simulink library "qrd_matrix_library"  (Simulink 8.7)
settings: Solver=ode45  StartTime=0.0  StopTime=10.0  RelTol=1e-3
values from neighbouring files (symbols this model uses):
  vectorization = 2    [qrd_test.m]
undefined symbols (not defined in the file or in its folder): AdvDSPBChannelOutDisplay, AdvDSPBDMemDisplay, Back_Substitution_instances, column_count, column_count_1, column_count_2, dpoly, dspba_ChannelInVis, dspba_ChannelOutVis, dspba_internal_get_channel_ports, evalAionMaskParam, latency, primtype, QRD_vectorization, recipsqrt, row, row_count, row_count_1, row_count_2, UseDontCare, value, x
libraries: DSPBAPrim x683, DSPBAControl x37, qrd_matrix_library x33, DSPBAVectorUtil x6, DSPBAVectorPrim x3
(part 2 of 8)

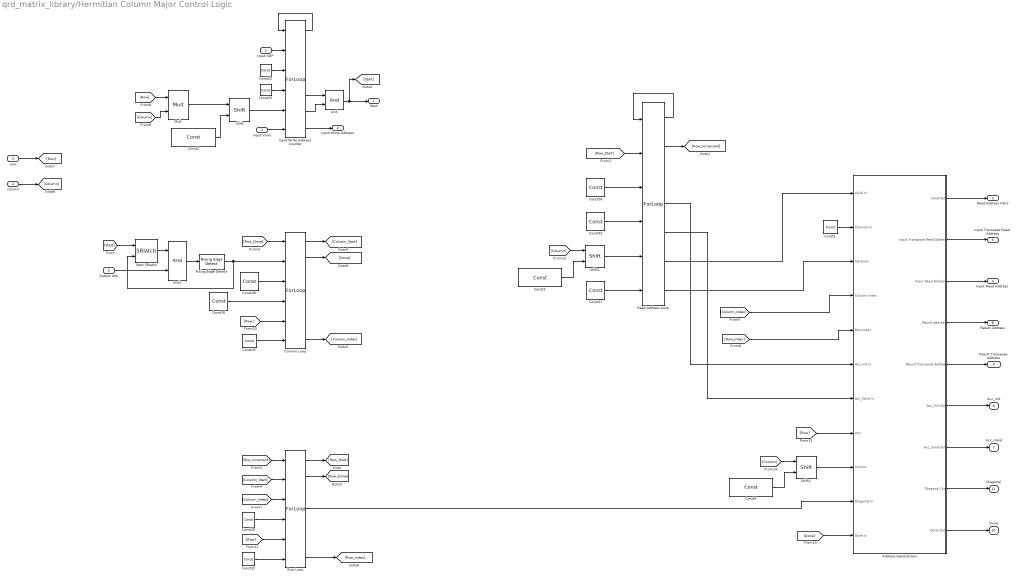
== system qrd_matrix_library/Hermitian Column Major Control Logic ==
  Input Valid : Inport
  Input SOP : Inport  Port=2
  row : Inport  Port=3
  column : Inport  Port=4
  Output Idle : Inport  Port=5
  Address Generatioon : Subsystem
  And : DSPBAPrim/And  primtype=and  nInputs=2  nOutputs=1  omode=Inherit via internal rule  otype=sfix(16)  scale=2^-15  rndmethod=Unbiased  factor=1  satmethod=Symmetric  shift_vec=[0 1 2 -1]  value=0  inPortNames=[' '; ' '; ' '; ' '; ' '; ' '; ' '; ' '; ' '; ' '; ' '; ' '; ' '; ' '; ' '; ' '; ]  outPortNames=[' ']  dspbaimage=dspba_prim.jpg  text=fprintf('&');  style=Optimised  visibilities=8+2  version=20090407
  And1 : DSPBAPrim/And  primtype=and  nInputs=2  nOutputs=1  omode=Inherit via internal rule  otype=sfix(16)  scale=2^-15  rndmethod=Unbiased  factor=1  satmethod=Symmetric  shift_vec=[0 1 2 -1]  value=0  inPortNames=[' '; ' '; ' '; ' '; ' '; ' '; ' '; ' '; ' '; ' '; ' '; ' '; ' '; ' '; ' '; ' '; ]  outPortNames=[' ']  dspbaimage=dspba_prim.jpg  text=fprintf('&');  style=Optimised  visibilities=8+2  version=20090407
  Column Loop : DSPBAPrim/ForLoop  looptest=<
  Const1 : DSPBAPrim/Const  primtype=const  nInputs=0  nOutputs=1  omode=Specify via dialog  otype=uint(8)  scale=1  rndmethod=Unbiased  factor=1  satmethod=Symmetric  shift_vec=[0 1 2 -1]  value=0  inPortNames=['+'; '+';]  outPortNames=[' ']  dspbaimage=dspba_prim.jpg  text=fprintf('%s', num2str(value));  style=Optimised  visibilities=8 + 1024  floatPrecision=float32_m23  version=20120820
  Const2 : DSPBAPrim/Const  primtype=const  nInputs=0  nOutputs=1  omode=Inherit via internal rule  otype=uint(8)  scale=1  rndmethod=Unbiased  factor=1  satmethod=Symmetric  shift_vec=[0 1 2 -1]  value=nextpow2(vectorization)  inPortNames=['+'; '+';]  outPortNames=[' ']  dspbaimage=dspba_prim.jpg  text=fprintf('%s', num2str(value));  style=Optimised  visibilities=8 + 1024  floatPrecision=float32_m23  version=20120820
  Const{23,26,29,33,35,37} (6 alike) : DSPBAPrim/Const  primtype=const  nInputs=0  nOutputs=1  omode=Inherit via internal rule  otype=uint(8)  scale=1  rndmethod=Unbiased  factor=1  satmethod=Symmetric  shift_vec=[0 1 2 -1]  value=1  inPortNames=['+'; '+';]  outPortNames=[' ']  dspbaimage=dspba_prim.jpg  text=fprintf('%s', num2str(value));  style=Optimised  visibilities=8 + 1024  floatPrecision=float32_m23  version=20120820
  Const25 : DSPBAPrim/Const  primtype=const  nInputs=0  nOutputs=1  omode=Inherit via internal rule  otype=uint(8)  scale=1  rndmethod=Unbiased  factor=1  satmethod=Symmetric  shift_vec=[0 1 2 -1]  value=0  inPortNames=['+'; '+';]  outPortNames=[' ']  dspbaimage=dspba_prim.jpg  text=fprintf('%s', num2str(value));  style=Optimised  visibilities=8 + 1024  floatPrecision=float32_m23  version=20120820
  Const28 : DSPBAPrim/Const  primtype=const  nInputs=0  nOutputs=1  omode=Inherit via internal rule  otype=uint(8)  scale=1  rndmethod=Unbiased  factor=1  satmethod=Symmetric  shift_vec=[0 1 2 -1]  value=0  inPortNames=['+'; '+';]  outPortNames=[' ']  dspbaimage=dspba_prim.jpg  text=fprintf('%s', num2str(value));  style=Optimised  visibilities=8 + 1024  floatPrecision=float32_m23  version=20120820
  Const3 : DSPBAPrim/Const  primtype=const  nInputs=0  nOutputs=1  omode=Inherit via internal rule  otype=uint(8)  scale=1  rndmethod=Unbiased  factor=1  satmethod=Symmetric  shift_vec=[0 1 2 -1]  value=nextpow2(vectorization)  inPortNames=['+'; '+';]  outPortNames=[' ']  dspbaimage=dspba_prim.jpg  text=fprintf('%s', num2str(value));  style=Optimised  visibilities=8 + 1024  floatPrecision=float32_m23  version=20120820
  Const32 : DSPBAPrim/Const  primtype=const  nInputs=0  nOutputs=1  omode=boolean  otype=uint(8)  scale=1  rndmethod=Unbiased  factor=1  satmethod=Symmetric  shift_vec=[0 1 2 -1]  value=1  inPortNames=['+'; '+';]  outPortNames=[' ']  dspbaimage=dspba_prim.jpg  text=fprintf('%s', num2str(value));  style=Optimised  visibilities=8 + 1024  floatPrecision=float32_m23  version=20120820
  Const36 : DSPBAPrim/Const  primtype=const  nInputs=0  nOutputs=1  omode=Inherit via internal rule  otype=uint(8)  scale=1  rndmethod=Unbiased  factor=1  satmethod=Symmetric  shift_vec=[0 1 2 -1]  value=0  inPortNames=['+'; '+';]  outPortNames=[' ']  dspbaimage=dspba_prim.jpg  text=fprintf('%s', num2str(value));  style=Optimised  visibilities=8 + 1024  floatPrecision=float32_m23  version=20120820
  Const4 : DSPBAPrim/Const  primtype=const  nInputs=0  nOutputs=1  omode=Inherit via internal rule  otype=uint(8)  scale=1  rndmethod=Unbiased  factor=1  satmethod=Symmetric  shift_vec=[0 1 2 -1]  value=nextpow2(vectorization)  inPortNames=['+'; '+';]  outPortNames=[' ']  dspbaimage=dspba_prim.jpg  text=fprintf('%s', num2str(value));  style=Optimised  visibilities=8 + 1024  floatPrecision=float32_m23  version=20120820
  Input Write Address Counter : DSPBAPrim/ForLoop  looptest=<
  Mult : DSPBAPrim/Mult  primtype=mult  nInputs=2  nOutputs=1  omode=Inherit via internal rule  otype=sfix(16)  scale=2^-15  rndmethod=Unbiased  factor=1  satmethod=Symmetric  shift_vec=[0 1 2 -1]  value=0  inPortNames=[' '; ' ';]  outPortNames=[' ']  dspbaimage=dspba_prim.jpg  text=fprintf('X');  style=Optimised  visibilities=8+2^18+2^19  floatPrecision=float32_m23  floatRounding=correct  advOptions=[]  version=20130115
  Read Address Loop : DSPBAPrim/ForLoop  looptest=<
  Rising Edge Detect : qrd_matrix_library/hermitian_matrix_multiplication/Rising Edge Detect
  Row Loop : DSPBAPrim/ForLoop  looptest=<
  Shift : DSPBAPrim/Shift  primtype=shift  nInputs=2  nOutputs=1  omode=Inherit via internal rule  otype=sfix(16)  scale=2^-15  rndmethod=Unbiased  factor=1  satmethod=Symmetric  shift_vec=[0 1 2 -1]  value=0  inPortNames=['a'; 'b';]  outPortNames=[' ']  dspbaimage=dspba_prim.jpg  text=fprintf('a >> b');  style=Optimised  visibilities=8  version=20090407
  Shift1 : DSPBAPrim/Shift  primtype=shift  nInputs=2  nOutputs=1  omode=Inherit via internal rule  otype=sfix(16)  scale=2^-15  rndmethod=Unbiased  factor=1  satmethod=Symmetric  shift_vec=[0 1 2 -1]  value=0  inPortNames=['a'; 'b';]  outPortNames=[' ']  dspbaimage=dspba_prim.jpg  text=fprintf('a >> b');  style=Optimised  visibilities=8  version=20090407
  Shift2 : DSPBAPrim/Shift  primtype=shift  nInputs=2  nOutputs=1  omode=Inherit via internal rule  otype=sfix(16)  scale=2^-15  rndmethod=Unbiased  factor=1  satmethod=Symmetric  shift_vec=[0 1 2 -1]  value=0  inPortNames=['a'; 'b';]  outPortNames=[' ']  dspbaimage=dspba_prim.jpg  text=fprintf('a >> b');  style=Optimised  visibilities=8  version=20090407
  Start SRlatch : DSPBAControl/SRlatch
  Start : Outport
  Input Write Address : Outport  Port=2
  Read Address Valid : Outport  Port=3
  Input Read Address : Outport  Port=4
  Input Transpose Read Address : Outport  Port=5
  Acc_Init : Outport  Port=6
  Acc_Valid : Outport  Port=7
  Result Address : Outport  Port=8
  Result Transpose Address : Outport  Port=9
  Done : Outport  Port=10
  Diagonal : Outport  Port=11
  wires:
  Address Generatioon/9(Done Out) -> Done/1
  [Done] -> Address Generatioon/11(Done In)
  [Row_Start] -> Read Address Loop/2
  Input SOP/1 -> Input Write Address Counter/2
  Read Address Loop/2 -> [Row_Increment]
  Input Write Address Counter/6 -> And/2
  Input Write Address Counter/5 -> And/1
  And/1 -> Start/1, [Start]
  Input Write Address Counter/1 -> Input Write Address Counter/1
  Input Valid/1 -> Input Write Address Counter/6
  Shift2/1 -> Address Generatioon/9(column)
  Const4/1 -> Shift2/2
  [Column] -> Shift2/1
  [Row] -> Address Generatioon/8(row)
  Const3/1 -> Shift1/2
  [Column] -> Shift1/1
  Const2/1 -> Shift/2
  Mult/1 -> Shift/1
  [Column] -> Mult/2
  [Row] -> Mult/1
  column/1 -> [Column]
  row/1 -> [Row]
  Address Generatioon/8(Diagonal Out) -> Diagonal/1
  Row Loop/4 -> Address Generatioon/10(Diagonal In)
  Const1/1 -> Address Generatioon/2(Channel In)
  Address Generatioon/6(Acc_Init Out) -> Acc_Init/1
  Address Generatioon/7(Acc_Valid Out) -> Acc_Valid/1
  Read Address Loop/6 -> Address Generatioon/1(Valid In)
  Address Generatioon/5(Result Transpose Address) -> Result Transpose Address/1
  Address Generatioon/4(Result Address) -> Result Address/1
  Address Generatioon/3(Input Read Address) -> Input Read Address/1
  Address Generatioon/2(Input Transpose Read Address) -> Input Transpose Read Address/1
  [Row_Index] -> Address Generatioon/5(Row Index)
  [Column_Index] -> Address Generatioon/4(Column Index)
  Read Address Loop/7 -> Address Generatioon/3(Iteration)
  Column Loop/2 -> [Done]
  Read Address Loop/5 -> Address Generatioon/7(Acc_Valid In)
  Read Address Loop/4 -> Address Generatioon/6(Acc_Init In)
  Address Generatioon/1(Valid Out) -> Read Address Valid/1
  Row Loop/7 -> [Row_Index]
  Const37/1 -> Read Address Loop/6
  Column Loop/1 -> [Column_Start]
  [Column_Start] -> Row Loop/2
  [Row_Done] -> Column Loop/1
  Row Loop/2 -> [Row_Done]
  [Row_Increment] -> Row Loop/1
  Row Loop/1 -> [Row_Start]
  Const35/1 -> Column Loop/6
  Const32/1 -> Row Loop/6
  Shift1/1 -> Read Address Loop/5
  Const33/1 -> Read Address Loop/4
  Const36/1 -> Read Address Loop/3
  Read Address Loop/1 -> Read Address Loop/1
  Column Loop/7 -> [Column_Index]
  [Column_Index] -> Row Loop/3
  Const29/1 -> Row Loop/4
  [Row] -> Row Loop/5
  Const28/1 -> Column Loop/3
  Const26/1 -> Column Loop/4
  [Row] -> Column Loop/5
  Input Write Address Counter/7 -> Input Write Address/1
  Const25/1 -> Input Write Address Counter/3
  Const23/1 -> Input Write Address Counter/4
  Shift/1 -> Input Write Address Counter/5
  [Start] -> Start SRlatch/1
  Start SRlatch/1 -> And1/1
  Output Idle/1 -> And1/2
  And1/1 -> Rising Edge Detect/1
  Rising Edge Detect/1 -> Column Loop/2, Start SRlatch/2

== system qrd_matrix_library/Hermitian Control Logic ==
  Input Valid : Inport
  Input SOP : Inport  Port=2
  row : Inport  Port=3
  column : Inport  Port=4
  Hermitian Column Major Control Logic : qrd_matrix_library/Hermitian Column Major Control Logic
  Start : Outport
  Input Write Address : Outport  Port=2
  Read Address Valid : Outport  Port=3
  Input Read Address : Outport  Port=4
  Input Transpose Read Address : Outport  Port=5
  Acc_Init : Outport  Port=6
  Acc_Valid : Outport  Port=7
  Result Address : Outport  Port=8
  Result Transpose Address : Outport  Port=9
  Done : Outport  Port=10
  Diagonal : Outport  Port=11
  wires:
  Input Valid/1 -> Hermitian Column Major Control Logic/1
  Input SOP/1 -> Hermitian Column Major Control Logic/2
  row/1 -> Hermitian Column Major Control Logic/3
  column/1 -> Hermitian Column Major Control Logic/4
  Hermitian Column Major Control Logic/1 -> Start/1
  Hermitian Column Major Control Logic/2 -> Input Write Address/1
  Hermitian Column Major Control Logic/3 -> Read Address Valid/1
  Hermitian Column Major Control Logic/4 -> Input Read Address/1
  Hermitian Column Major Control Logic/5 -> Input Transpose Read Address/1
  Hermitian Column Major Control Logic/6 -> Acc_Init/1
  Hermitian Column Major Control Logic/7 -> Acc_Valid/1
  Hermitian Column Major Control Logic/8 -> Result Address/1
  Hermitian Column Major Control Logic/9 -> Result Transpose Address/1
  Hermitian Column Major Control Logic/10 -> Done/1
  Hermitian Column Major Control Logic/11 -> Diagonal/1

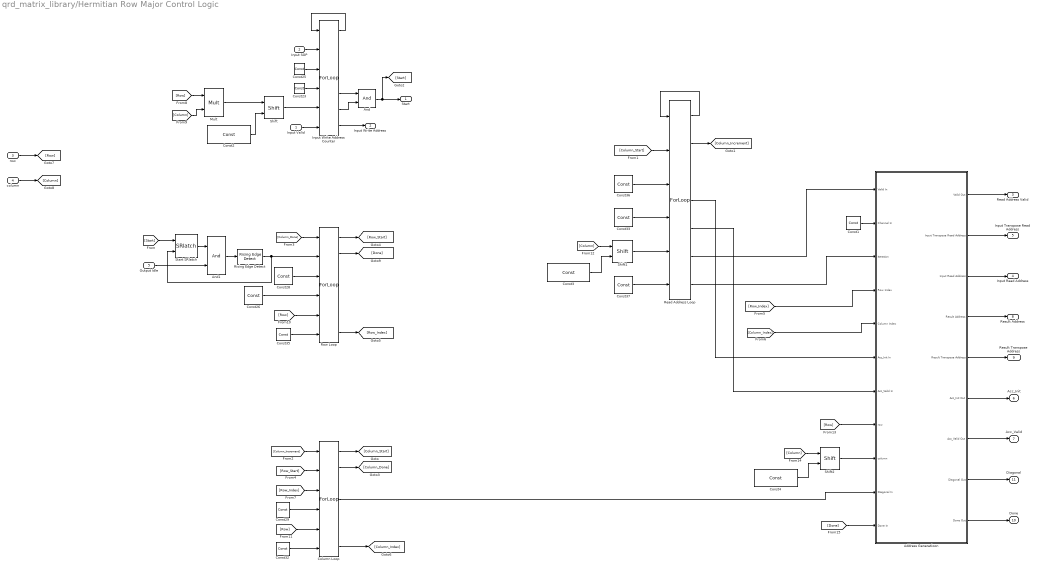
== system qrd_matrix_library/Hermitian Row Major Control Logic ==
  Input Valid : Inport
  Input SOP : Inport  Port=2
  row : Inport  Port=3
  column : Inport  Port=4
  Output Idle : Inport  Port=5
  Address Generatioon : Subsystem
  And : DSPBAPrim/And  primtype=and  nInputs=2  nOutputs=1  omode=Inherit via internal rule  otype=sfix(16)  scale=2^-15  rndmethod=Unbiased  factor=1  satmethod=Symmetric  shift_vec=[0 1 2 -1]  value=0  inPortNames=[' '; ' '; ' '; ' '; ' '; ' '; ' '; ' '; ' '; ' '; ' '; ' '; ' '; ' '; ' '; ' '; ]  outPortNames=[' ']  dspbaimage=dspba_prim.jpg  text=fprintf('&');  style=Optimised  visibilities=8+2  version=20090407
  And1 : DSPBAPrim/And  primtype=and  nInputs=2  nOutputs=1  omode=Inherit via internal rule  otype=sfix(16)  scale=2^-15  rndmethod=Unbiased  factor=1  satmethod=Symmetric  shift_vec=[0 1 2 -1]  value=0  inPortNames=[' '; ' '; ' '; ' '; ' '; ' '; ' '; ' '; ' '; ' '; ' '; ' '; ' '; ' '; ' '; ' '; ]  outPortNames=[' ']  dspbaimage=dspba_prim.jpg  text=fprintf('&');  style=Optimised  visibilities=8+2  version=20090407
  Column Loop : DSPBAPrim/ForLoop  looptest=<
  Const1 : DSPBAPrim/Const  primtype=const  nInputs=0  nOutputs=1  omode=Specify via dialog  otype=uint(8)  scale=1  rndmethod=Unbiased  factor=1  satmethod=Symmetric  shift_vec=[0 1 2 -1]  value=0  inPortNames=['+'; '+';]  outPortNames=[' ']  dspbaimage=dspba_prim.jpg  text=fprintf('%s', num2str(value));  style=Optimised  visibilities=8 + 1024  floatPrecision=float32_m23  version=20120820
  Const2 : DSPBAPrim/Const  primtype=const  nInputs=0  nOutputs=1  omode=Inherit via internal rule  otype=uint(8)  scale=1  rndmethod=Unbiased  factor=1  satmethod=Symmetric  shift_vec=[0 1 2 -1]  value=nextpow2(vectorization)  inPortNames=['+'; '+';]  outPortNames=[' ']  dspbaimage=dspba_prim.jpg  text=fprintf('%s', num2str(value));  style=Optimised  visibilities=8 + 1024  floatPrecision=float32_m23  version=20120820
  Const{23,26,29,33,35,37} (6 alike) : DSPBAPrim/Const  primtype=const  nInputs=0  nOutputs=1  omode=Inherit via internal rule  otype=uint(8)  scale=1  rndmethod=Unbiased  factor=1  satmethod=Symmetric  shift_vec=[0 1 2 -1]  value=1  inPortNames=['+'; '+';]  outPortNames=[' ']  dspbaimage=dspba_prim.jpg  text=fprintf('%s', num2str(value));  style=Optimised  visibilities=8 + 1024  floatPrecision=float32_m23  version=20120820
  Const25 : DSPBAPrim/Const  primtype=const  nInputs=0  nOutputs=1  omode=Inherit via internal rule  otype=uint(8)  scale=1  rndmethod=Unbiased  factor=1  satmethod=Symmetric  shift_vec=[0 1 2 -1]  value=0  inPortNames=['+'; '+';]  outPortNames=[' ']  dspbaimage=dspba_prim.jpg  text=fprintf('%s', num2str(value));  style=Optimised  visibilities=8 + 1024  floatPrecision=float32_m23  version=20120820
  Const28 : DSPBAPrim/Const  primtype=const  nInputs=0  nOutputs=1  omode=Inherit via internal rule  otype=uint(8)  scale=1  rndmethod=Unbiased  factor=1  satmethod=Symmetric  shift_vec=[0 1 2 -1]  value=0  inPortNames=['+'; '+';]  outPortNames=[' ']  dspbaimage=dspba_prim.jpg  text=fprintf('%s', num2str(value));  style=Optimised  visibilities=8 + 1024  floatPrecision=float32_m23  version=20120820
  Const3 : DSPBAPrim/Const  primtype=const  nInputs=0  nOutputs=1  omode=Inherit via internal rule  otype=uint(8)  scale=1  rndmethod=Unbiased  factor=1  satmethod=Symmetric  shift_vec=[0 1 2 -1]  value=nextpow2(vectorization)  inPortNames=['+'; '+';]  outPortNames=[' ']  dspbaimage=dspba_prim.jpg  text=fprintf('%s', num2str(value));  style=Optimised  visibilities=8 + 1024  floatPrecision=float32_m23  version=20120820
  Const32 : DSPBAPrim/Const  primtype=const  nInputs=0  nOutputs=1  omode=boolean  otype=uint(8)  scale=1  rndmethod=Unbiased  factor=1  satmethod=Symmetric  shift_vec=[0 1 2 -1]  value=1  inPortNames=['+'; '+';]  outPortNames=[' ']  dspbaimage=dspba_prim.jpg  text=fprintf('%s', num2str(value));  style=Optimised  visibilities=8 + 1024  floatPrecision=float32_m23  version=20120820
  Const36 : DSPBAPrim/Const  primtype=const  nInputs=0  nOutputs=1  omode=Inherit via internal rule  otype=uint(8)  scale=1  rndmethod=Unbiased  factor=1  satmethod=Symmetric  shift_vec=[0 1 2 -1]  value=0  inPortNames=['+'; '+';]  outPortNames=[' ']  dspbaimage=dspba_prim.jpg  text=fprintf('%s', num2str(value));  style=Optimised  visibilities=8 + 1024  floatPrecision=float32_m23  version=20120820
  Const4 : DSPBAPrim/Const  primtype=const  nInputs=0  nOutputs=1  omode=Inherit via internal rule  otype=uint(8)  scale=1  rndmethod=Unbiased  factor=1  satmethod=Symmetric  shift_vec=[0 1 2 -1]  value=nextpow2(vectorization)  inPortNames=['+'; '+';]  outPortNames=[' ']  dspbaimage=dspba_prim.jpg  text=fprintf('%s', num2str(value));  style=Optimised  visibilities=8 + 1024  floatPrecision=float32_m23  version=20120820
  Input Write Address Counter : DSPBAPrim/ForLoop  looptest=<
  Mult : DSPBAPrim/Mult  primtype=mult  nInputs=2  nOutputs=1  omode=Inherit via internal rule  otype=sfix(16)  scale=2^-15  rndmethod=Unbiased  factor=1  satmethod=Symmetric  shift_vec=[0 1 2 -1]  value=0  inPortNames=[' '; ' ';]  outPortNames=[' ']  dspbaimage=dspba_prim.jpg  text=fprintf('X');  style=Optimised  visibilities=8+2^18+2^19  floatPrecision=float32_m23  floatRounding=correct  advOptions=[]  version=20130115
  Read Address Loop : DSPBAPrim/ForLoop  looptest=<
  Rising Edge Detect : qrd_matrix_library/hermitian_matrix_multiplication/Rising Edge Detect
  Row Loop : DSPBAPrim/ForLoop  looptest=<
  Shift : DSPBAPrim/Shift  primtype=shift  nInputs=2  nOutputs=1  omode=Inherit via internal rule  otype=sfix(16)  scale=2^-15  rndmethod=Unbiased  factor=1  satmethod=Symmetric  shift_vec=[0 1 2 -1]  value=0  inPortNames=['a'; 'b';]  outPortNames=[' ']  dspbaimage=dspba_prim.jpg  text=fprintf('a >> b');  style=Optimised  visibilities=8  version=20090407
  Shift1 : DSPBAPrim/Shift  primtype=shift  nInputs=2  nOutputs=1  omode=Inherit via internal rule  otype=sfix(16)  scale=2^-15  rndmethod=Unbiased  factor=1  satmethod=Symmetric  shift_vec=[0 1 2 -1]  value=0  inPortNames=['a'; 'b';]  outPortNames=[' ']  dspbaimage=dspba_prim.jpg  text=fprintf('a >> b');  style=Optimised  visibilities=8  version=20090407
  Shift2 : DSPBAPrim/Shift  primtype=shift  nInputs=2  nOutputs=1  omode=Inherit via internal rule  otype=sfix(16)  scale=2^-15  rndmethod=Unbiased  factor=1  satmethod=Symmetric  shift_vec=[0 1 2 -1]  value=0  inPortNames=['a'; 'b';]  outPortNames=[' ']  dspbaimage=dspba_prim.jpg  text=fprintf('a >> b');  style=Optimised  visibilities=8  version=20090407
  Start SRlatch : DSPBAControl/SRlatch
  Start : Outport
  Input Write Address : Outport  Port=2
  Read Address Valid : Outport  Port=3
  Input Read Address : Outport  Port=4
  Input Transpose Read Address : Outport  Port=5
  Acc_Init : Outport  Port=6
  Acc_Valid : Outport  Port=7
  Result Address : Outport  Port=8
  Result Transpose Address : Outport  Port=9
  Done : Outport  Port=10
  Diagonal : Outport  Port=11
  wires:
  Address Generatioon/9(Done Out) -> Done/1
  [Done] -> Address Generatioon/11(Done In)
  [Column_Start] -> Read Address Loop/2
  Input SOP/1 -> Input Write Address Counter/2
  Read Address Loop/2 -> [Column_Increment]
  Input Write Address Counter/6 -> And/2
  Input Write Address Counter/5 -> And/1
  And/1 -> Start/1, [Start]
  Input Write Address Counter/1 -> Input Write Address Counter/1
  Input Valid/1 -> Input Write Address Counter/6
  Shift2/1 -> Address Generatioon/9(column)
  Const4/1 -> Shift2/2
  [Column] -> Shift2/1
  [Row] -> Address Generatioon/8(row)
  Const3/1 -> Shift1/2
  [Column] -> Shift1/1
  Const2/1 -> Shift/2
  Mult/1 -> Shift/1
  [Column] -> Mult/2
  [Row] -> Mult/1
  column/1 -> [Column]
  row/1 -> [Row]
  Address Generatioon/8(Diagonal Out) -> Diagonal/1
  Column Loop/4 -> Address Generatioon/10(Diagonal In)
  Const1/1 -> Address Generatioon/2(Channel In)
  Address Generatioon/6(Acc_Init Out) -> Acc_Init/1
  Address Generatioon/7(Acc_Valid Out) -> Acc_Valid/1
  Read Address Loop/6 -> Address Generatioon/1(Valid In)
  Address Generatioon/5(Result Transpose Address) -> Result Transpose Address/1
  Address Generatioon/4(Result Address) -> Result Address/1
  Address Generatioon/3(Input Read Address) -> Input Read Address/1
  Address Generatioon/2(Input Transpose Read Address) -> Input Transpose Read Address/1
  [Column_Index] -> Address Generatioon/5(Column Index)
  [Row_Index] -> Address Generatioon/4(Row Index)
  Read Address Loop/7 -> Address Generatioon/3(Iteration)
  Row Loop/2 -> [Done]
  Read Address Loop/5 -> Address Generatioon/7(Acc_Valid In)
  Read Address Loop/4 -> Address Generatioon/6(Acc_Init In)
  Address Generatioon/1(Valid Out) -> Read Address Valid/1
  Column Loop/7 -> [Column_Index]
  Const37/1 -> Read Address Loop/6
  Row Loop/1 -> [Row_Start]
  [Row_Start] -> Column Loop/2
  [Column_Done] -> Row Loop/1
  Column Loop/2 -> [Column_Done]
  [Column_Increment] -> Column Loop/1
  Column Loop/1 -> [Column_Start]
  Const35/1 -> Row Loop/6
  Const32/1 -> Column Loop/6
  Shift1/1 -> Read Address Loop/5
  Const33/1 -> Read Address Loop/4
  Const36/1 -> Read Address Loop/3
  Read Address Loop/1 -> Read Address Loop/1
  Row Loop/7 -> [Row_Index]
  [Start] -> Start SRlatch/1
  [Row_Index] -> Column Loop/3
  Const29/1 -> Column Loop/4
  [Row] -> Column Loop/5
  Const28/1 -> Row Loop/3
  Const26/1 -> Row Loop/4
  [Row] -> Row Loop/5
  Input Write Address Counter/7 -> Input Write Address/1
  Const25/1 -> Input Write Address Counter/3
  Const23/1 -> Input Write Address Counter/4
  Shift/1 -> Input Write Address Counter/5
  Start SRlatch/1 -> And1/1
  Output Idle/1 -> And1/2
  And1/1 -> Rising Edge Detect/1
  Rising Edge Detect/1 -> Start SRlatch/2, Row Loop/2

== system qrd_matrix_library/Latch ==
  Valid_In : Inport
  Channel_In : Inport  Port=2
  Data_In : Inport  Port=3
  ChannelIn : DSPBAPrim/ChannelIn  primtype=channelin  nInputs=dspba_internal_get_channel_ports(gcb)  nOutputs=dspba_internal_get_channel_ports(gcb)  omode=Inherit via internal rule  otype=sfix(16)  scale=2^-15  rndmethod=Unbiased  factor=1  satmethod=Symmetric  shift_vec=[0 1 2 -1]  value=1  inPortNames=['v'; 'c'; '0'; '1'; '2'; '3'; '4'; '5'; '6'; '7'; '8'; '9'; 'A'; 'B'; 'D'; 'E'; 'F'; 'G'; 'H'; 'I'; 'J'; 'K'; 'L'; 'M'; 'N'; 'O'; 'P'; 'Q'; 'R'; 'S'; 'T'; 'U'; 'W'; 'X'; 'Y'; 'Z']  outPortNames=['v'; 'c'; '0'; '1'; '2'; '3'; '4'; '5'; '6'; '7'; '8'; '9'; 'A'; 'B'; 'D'; 'E'; 'F'; 'G'; 'H'; 'I'; 'J'; 'K'; 'L'; 'M'; 'N'; 'O'; 'P'; 'Q'; 'R'; 'S'; 'T'; 'U'; 'W'; 'X'; 'Y'; 'Z']  dspbaimage=dspba_prim.jpg  text=fprintf('In');  style=Optimised  dataSignals=1  foldingEnabled=off  channels=1  sampleRate=200  packetBeginPresent=off  packetBeginEnabled=off  visibilities=dspba_ChannelInVis(gcb)  latencyCorrection=0  version=20141013
  ChannelOut : DSPBAPrim/ChannelOut  primtype=channelout  nInputs=dspba_internal_get_channel_ports(gcb)  nOutputs=dspba_internal_get_channel_ports(gcb)  omode=Inherit via internal rule  otype=sfix(16)  scale=2^-15  rndmethod=Unbiased  factor=1  satmethod=Symmetric  shift_vec=[0 1 2 -1]  value=1  inPortNames=['v'; 'c'; '0'; '1'; '2'; '3'; '4'; '5'; '6'; '7'; '8'; '9'; 'A'; 'B'; 'D'; 'E'; 'F'; 'G'; 'H'; 'I'; 'J'; 'K'; 'L'; 'M'; 'N'; 'O'; 'P'; 'Q'; 'R'; 'S'; 'T'; 'U'; 'W'; 'X'; 'Y'; 'Z']  outPortNames=['v'; 'c'; '0'; '1'; '2'; '3'; '4'; '5'; '6'; '7'; '8'; '9'; 'A'; 'B'; 'D'; 'E'; 'F'; 'G'; 'H'; 'I'; 'J'; 'K'; 'L'; 'M'; 'N'; 'O'; 'P'; 'Q'; 'R'; 'S'; 'T'; 'U'; 'W'; 'X'; 'Y'; 'Z']  dspbaimage=dspba_prim.jpg  text=fprintf('Out%s', AdvDSPBChannelOutDisplay(latency));  style=Optimised  dataSignals=1  foldingEnabled=off  channels=1  sampleRate=200  packetBeginPresent=off  packetBeginEnabled=off  visibilities=dspba_ChannelOutVis(gcb)  latency=0  latencyCorrection=0  version=20141013
  SynthesisInfo : DSPBAPrim/SynthesisInfo  primtype=synthinfo  nInputs=0  nOutputs=0  omode=Inherit via internal rule  otype=sfix(16)  scale=2^-15  rndmethod=Truncate  factor=1  satmethod=Symmetric  shift_vec=[0 1 2 -1]  value=99  inPortNames=[' '; ' ';]  outPortNames=[' ']  dspbaimage=dspba_prim_ctrl.jpg  text=fprintf('Style=%s', style);  style=Scheduled  visibilities=32768  constraintInUse=off  constraintRelation=>  constraintLimit=2  bitAccurate=off  version=20150220
  latch_0L : DSPBAControl/latch_0L
  Valid_Out : Outport
  Channel_Out : Outport  Port=2
  Data_Out : Outport  Port=3
  wires:
  Valid_In/1 -> ChannelIn/1
  Data_In/1 -> ChannelIn/3
  Channel_In/1 -> ChannelIn/2
  ChannelIn/1 -> ChannelOut/1, latch_0L/1
  latch_0L/1 -> ChannelOut/3
  ChannelIn/2 -> ChannelOut/2
  ChannelIn/3 -> latch_0L/2
  ChannelOut/1 -> Valid_Out/1
  ChannelOut/3 -> Data_Out/1
  ChannelOut/2 -> Channel_Out/1

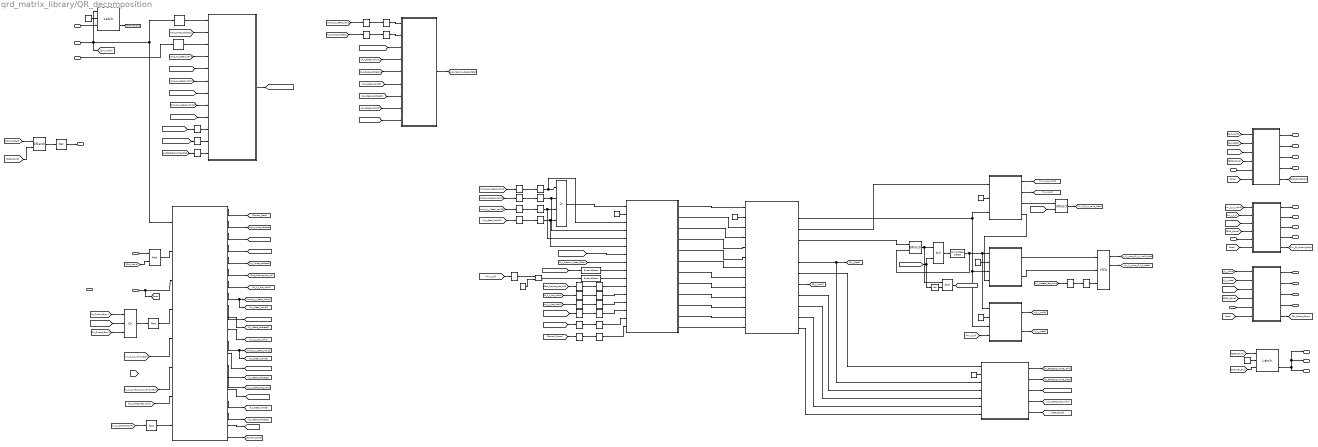
== system qrd_matrix_library/QR_decomposition ==
  Sink Valid : Inport
  Sink Channel : Inport  Port=2
  Sink Data : Inport  Port=3
  Sink SOP : Inport  Port=4
  Sink EOP : Inport  Port=5
  Q Source Ready : Inport  Port=6
  Inv Rk Source Ready : Inport  Port=7
  Rn Source Ready : Inport  Port=8
  size : Inport  Port=9
  A_j : Subsystem
  A_k Memory Controller : Subsystem
  Address Delay : DSPBAPrim/SampleDelay  primtype=sampdelay  nInputs=1  nOutputs=1  omode=Inherit via internal rule  otype=sfix(16)  scale=2^-15  rndmethod=Unbiased  factor=1  satmethod=Symmetric  shift_vec=[0 1 2 -1]  value=1  inPortNames=[' '; ' ';]  outPortNames=[' ']  dspbaimage=dspba_prim.jpg  text=dpoly(1, eye(1,value+1), 'z')  style=Optimised  visibilities=8 + 1024 + 2^17 + 2^18  flexible=off  slackgroup=0  augmented=0  version=20090407  advOptions=[]
  Address Delay1 : DSPBAPrim/SampleDelay  primtype=sampdelay  nInputs=1  nOutputs=1  omode=Inherit via internal rule  otype=sfix(16)  scale=2^-15  rndmethod=Unbiased  factor=1  satmethod=Symmetric  shift_vec=[0 1 2 -1]  value=1  inPortNames=[' '; ' ';]  outPortNames=[' ']  dspbaimage=dspba_prim.jpg  text=dpoly(1, eye(1,value+1), 'z')  style=Optimised  visibilities=8 + 1024 + 2^17 + 2^18  flexible=off  slackgroup=0  augmented=0  version=20090407  advOptions=[]
  And : DSPBAPrim/And  primtype=and  nInputs=2  nOutputs=1  omode=Inherit via internal rule  otype=sfix(16)  scale=2^-15  rndmethod=Unbiased  factor=1  satmethod=Symmetric  shift_vec=[0 1 2 -1]  value=0  inPortNames=[' '; ' '; ' '; ' '; ' '; ' '; ' '; ' '; ' '; ' '; ' '; ' '; ' '; ' '; ' '; ' '; ]  outPortNames=[' ']  dspbaimage=dspba_prim.jpg  text=fprintf('&');  style=Optimised  visibilities=8+2  version=20090407
  And4 : DSPBAPrim/And  primtype=and  nInputs=2  nOutputs=1  omode=Inherit via internal rule  otype=sfix(16)  scale=2^-15  rndmethod=Unbiased  factor=1  satmethod=Symmetric  shift_vec=[0 1 2 -1]  value=0  inPortNames=[' '; ' '; ' '; ' '; ' '; ' '; ' '; ' '; ' '; ' '; ' '; ' '; ' '; ' '; ' '; ' '; ]  outPortNames=[' ']  dspbaimage=dspba_prim.jpg  text=fprintf('&');  style=Optimised  visibilities=8+2  version=20090407
  Channel Latch : qrd_matrix_library/Latch
  Const11 : DSPBAPrim/Const  primtype=const  nInputs=0  nOutputs=1  omode=single  otype=uint(8)  scale=1  rndmethod=Unbiased  factor=1  satmethod=Symmetric  shift_vec=[0 1 2 -1]  value=0  inPortNames=['+'; '+';]  outPortNames=[' ']  dspbaimage=dspba_prim.jpg  text=fprintf('%s', num2str(value));  style=Optimised  visibilities=8 + 1024  floatPrecision=float32_m23  version=20120820
  Const{2..8,13} (8 alike) : DSPBAPrim/Const  primtype=const  nInputs=0  nOutputs=1  omode=Specify via dialog  otype=uint(8)  scale=1  rndmethod=Unbiased  factor=1  satmethod=Symmetric  shift_vec=[0 1 2 -1]  value=0  inPortNames=['+'; '+';]  outPortNames=[' ']  dspbaimage=dspba_prim.jpg  text=fprintf('%s', num2str(value));  style=Optimised  visibilities=8 + 1024  floatPrecision=float32_m23  version=20120820
  Control Logic : Subsystem
  Data Mux : Subsystem
  Data_Mux_Valid_Or : DSPBAPrim/Or  primtype=or  nInputs=4  nOutputs=1  omode=Inherit via internal rule  otype=sfix(16)  scale=2^-15  rndmethod=Unbiased  factor=1  satmethod=Symmetric  shift_vec=[0 1 2 -1]  value=0  inPortNames=[' '; ' '; ' '; ' '; ' '; ' '; ' '; ' '; ' '; ' '; ' '; ' '; ' '; ' '; ' '; ' '; ]  outPortNames=[' ']  dspbaimage=dspba_prim.jpg  text=fprintf('|');  style=Optimised  visibilities=8+2  version=20090407
  Dot Product : Subsystem
  ExpandScalar : DSPBAVectorUtil/ExpandScalar  vecWidth=vectorization
  ExpandScalar1 : DSPBAVectorUtil/ExpandScalar  vecWidth=vectorization
  Feedback delay : DSPBAPrim/SampleDelay  primtype=sampdelay  nInputs=1  nOutputs=1  omode=Inherit via internal rule  otype=sfix(16)  scale=2^-15  rndmethod=Unbiased  factor=1  satmethod=Symmetric  shift_vec=[0 1 2 -1]  value=1  inPortNames=[' '; ' ';]  outPortNames=[' ']  dspbaimage=dspba_prim.jpg  text=dpoly(1, eye(1,value+1), 'z')  style=Optimised  visibilities=8 + 1024 + 2^17 + 2^18  flexible=off  slackgroup=0  augmented=0  version=20090407  advOptions=[]
  Feedback delay1 : DSPBAPrim/SampleDelay  primtype=sampdelay  nInputs=1  nOutputs=1  omode=Inherit via internal rule  otype=sfix(16)  scale=2^-15  rndmethod=Unbiased  factor=1  satmethod=Symmetric  shift_vec=[0 1 2 -1]  value=1  inPortNames=[' '; ' ';]  outPortNames=[' ']  dspbaimage=dspba_prim.jpg  text=dpoly(1, eye(1,value+1), 'z')  style=Optimised  visibilities=8 + 1024 + 2^17 + 2^18  flexible=off  slackgroup=0  augmented=0  version=20090407  advOptions=[]
  Feedback delay2 : DSPBAPrim/SampleDelay  primtype=sampdelay  nInputs=1  nOutputs=1  omode=Inherit via internal rule  otype=sfix(16)  scale=2^-15  rndmethod=Unbiased  factor=1  satmethod=Symmetric  shift_vec=[0 1 2 -1]  value=1  inPortNames=[' '; ' ';]  outPortNames=[' ']  dspbaimage=dspba_prim.jpg  text=dpoly(1, eye(1,value+1), 'z')  style=Optimised  visibilities=8 + 1024 + 2^17 + 2^18  flexible=off  slackgroup=0  augmented=0  version=20090407  advOptions=[]
  Input Memory Controller : Subsystem
  Inv SQRT : Subsystem
  Inv_Rk Output Memory Controller : Subsystem
  Latch : qrd_matrix_library/Latch
  Mem Address Select Delay{1..4,6..8,11..12} (9 alike) : DSPBAPrim/SampleDelay  primtype=sampdelay  nInputs=1  nOutputs=1  omode=Inherit via internal rule  otype=sfix(16)  scale=2^-15  rndmethod=Unbiased  factor=1  satmethod=Symmetric  shift_vec=[0 1 2 -1]  value=1  inPortNames=[' '; ' ';]  outPortNames=[' ']  dspbaimage=dspba_prim.jpg  text=dpoly(1, eye(1,value+1), 'z')  style=Optimised  visibilities=8 + 1024 + 2^17 + 2^18  flexible=off  slackgroup=0  augmented=0  version=20090407  advOptions=[]
  Memory Delay{1..13} (13 alike) : DSPBAPrim/SampleDelay  primtype=sampdelay  nInputs=1  nOutputs=1  omode=Inherit via internal rule  otype=sfix(16)  scale=2^-15  rndmethod=Unbiased  factor=1  satmethod=Symmetric  shift_vec=[0 1 2 -1]  value=2  inPortNames=[' '; ' ';]  outPortNames=[' ']  dspbaimage=dspba_prim.jpg  text=dpoly(1, eye(1,value+1), 'z')  style=Optimised  visibilities=8 + 1024 + 2^17 + 2^18  flexible=off  slackgroup=0  augmented=0  version=20090407  advOptions=[]
  Mux Delay{1..5} (5 alike) : DSPBAPrim/SampleDelay  primtype=sampdelay  nInputs=1  nOutputs=1  omode=Inherit via internal rule  otype=sfix(16)  scale=2^-15  rndmethod=Unbiased  factor=1  satmethod=Symmetric  shift_vec=[0 1 2 -1]  value=1  inPortNames=[' '; ' ';]  outPortNames=[' ']  dspbaimage=dspba_prim.jpg  text=dpoly(1, eye(1,value+1), 'z')  style=Optimised  visibilities=8 + 1024 + 2^17 + 2^18  flexible=off  slackgroup=0  augmented=0  version=20090407  advOptions=[]
  Not{,1..3} (4 alike) : DSPBAPrim/Not  primtype=not  nInputs=1  nOutputs=1  omode=Inherit via internal rule  otype=sfix(16)  scale=2^-15  rndmethod=Unbiased  factor=1  satmethod=Symmetric  shift_vec=[0 1 2 -1]  value=0  inPortNames=[' '; ' ';]  outPortNames=[' ']  dspbaimage=dspba_prim.jpg  text=fprintf('~');  style=Optimised  visibilities=8  version=20090407
  Or : DSPBAPrim/Or  primtype=or  nInputs=3  nOutputs=1  omode=Inherit via internal rule  otype=sfix(16)  scale=2^-15  rndmethod=Unbiased  factor=1  satmethod=Symmetric  shift_vec=[0 1 2 -1]  value=0  inPortNames=[' '; ' '; ' '; ' '; ' '; ' '; ' '; ' '; ' '; ' '; ' '; ' '; ' '; ' '; ' '; ' '; ]  outPortNames=[' ']  dspbaimage=dspba_prim.jpg  text=fprintf('|');  style=Optimised  visibilities=8+2  version=20090407
  Q Output Memory Controller : Subsystem
  Real-Imag to Complex : RealImagToComplex
  Rising Edge Detect3 : qrd_matrix_library/hermitian_matrix_multiplication/Rising Edge Detect
  Rn Output Memory Controller : Subsystem
  SOP_And : DSPBAPrim/And  primtype=and  nInputs=2  nOutputs=1  omode=Inherit via internal rule  otype=sfix(16)  scale=2^-15  rndmethod=Unbiased  factor=1  satmethod=Symmetric  shift_vec=[0 1 2 -1]  value=0  inPortNames=[' '; ' '; ' '; ' '; ' '; ' '; ' '; ' '; ' '; ' '; ' '; ' '; ' '; ' '; ' '; ' '; ]  outPortNames=[' ']  dspbaimage=dspba_prim.jpg  text=fprintf('&');  style=Optimised  visibilities=8+2  version=20090407
  Sink Ready SRlatch : DSPBAControl/SRlatch
  inv_r2_k_k SRlatch : DSPBAControl/SRlatch
  rk : Subsystem
  rn_k_j SRlatch : DSPBAControl/SRlatch
  rn_k_j_over_r2_k_k : Subsystem
  rn_k_j_over_r2_k_k FIFO : DSPBAPrim/FIFO  primtype=fifo  nInputs=3  nOutputs=4  omode=Inherit via internal rule  otype=sfix(16)  scale=2^-15  rndmethod=Unbiased  factor=1  satmethod=Symmetric  shift_vec=[0 1 2 -1]  value=[(size-1) 4 (size-1)]  inPortNames=['w'; 'd'; 'r'; 'f']  outPortNames=['v'; 'q'; 't'; 'f']  dspbaimage=dspba_prim.jpg  text=fprintf('fifo');  style=Optimised  visibilities=263168  version=20130808  user_sclr=off
  Sink Ready : Outport
  Q Source Valid : Outport  Port=2
  Q Source Channel : Outport  Port=3
  Q Source Data : Outport  Port=4
  Q Source SOP : Outport  Port=5
  Q Source EOP : Outport  Port=6
  Inv Rk Source Valid : Outport  Port=7
  Inv Rk Source Channel : Outport  Port=8
  Inv Rk Source Data : Outport  Port=9
  Inv Rk Source SOP : Outport  Port=10
  Inv Rk Source EOP : Outport  Port=11
  Rn Source Valid : Outport  Port=12
  Rn Source Channel : Outport  Port=13
  Rn Source Data : Outport  Port=14
  Rn Source SOP : Outport  Port=15
  Rn Source EOP : Outport  Port=16
  wires:
  Address Delay/1 -> Input Memory Controller/1(External Write)
  Sink Data/1 -> Address Delay1/1
  Control Logic/2(Input Write Address) -> [Input_Write_Address]
  Address Delay1/1 -> Input Memory Controller/3(External Write Data)
  [Input_Write_Address] -> Input Memory Controller/2(External Write Address)
  Sink SOP/1 -> SOP_And/1
  [Input_A_k_Read_Valid] -> Input Memory Controller/4(Input_A_k_Read_Valid)
  Sink Valid/1 -> [Sink_Valid], Control Logic/1(Input Valid), Address Delay/1, Latch/1
  size/1 -> [size], Control Logic/3(size)
  Not/1 -> Sink Ready/1
  [QRD_Done] -> Sink Ready SRlatch/2
  Sink Channel/1 -> Latch/3
  Const6/1 -> Latch/2
  Sink Ready SRlatch/1 -> Not/1
  [Sink_Valid] -> SOP_And/2
  SOP_And/1 -> Control Logic/2(Input SOP)
  Control Logic/1(Start) -> [Control_Start]
  [Control_Start] -> Sink Ready SRlatch/1
  Not1/1 -> Control Logic/4(Output Idle)
  Or/1 -> Not1/1
  Control Logic/3(Input_A_k_Read_Valid) -> [Input_A_k_Read_Valid]
  Control Logic/4(Input_A_k_Read_Address) -> [Input_A_k_Read_Address]
  [Input_A_k_Read_Address] -> Input Memory Controller/5(Input_A_k_Read_Address)
  [A_k_Write_Address] -> Mux Delay2/1
  [Input_A_k_Read_Valid] -> Mux Delay1/1
  Memory Delay3/1 -> A_k Memory Controller/2(Write_Address)
  Memory Delay4/1 -> A_k Memory Controller/1(Write_Enable)
  [Input_Memory_Read_Data] -> A_k Memory Controller/3(Write_Data)
  A_k Memory Controller/1(Read_Data) -> [A_k_Memory_Read_Data]
  Input Memory Controller/1(Read Data) -> [Input_Memory_Read_Data]
  Control Logic/5(A_k_Write_Address) -> [A_k_Write_Address]
  Control Logic/6(Dot_Product_Init) -> [Dot_Product_Acc_Init]
  Control Logic/7(r2_k_k_acc_valid) -> [r2_k_k_Acc_Valid]
  Const3/1 -> Dot Product/2(Channel_In)
  Data Mux/4(Dot_Product_Acc_Init_Out) -> Dot Product/5(Acc_Init)
  Dot Product/3(r2_k_k_valid_out) -> Inv SQRT/1(Valid In)
  [r2_k_k_Acc_Valid] -> Mux Delay5/1
  [Dot_Product_Acc_Init] -> Mux Delay4/1
  Control Logic/8(Input_A_j_Read_Valid1) -> [A_k_Read_Valid1], [Input_A_j_Read_Valid1]
  Control Logic/9(Input_A_j_Read_Address1) -> [Input_A_j_Read_Address1]
  Control Logic/10(A_k_Read_Address1) -> [A_k_Read_Address1]
  Control Logic/11(rn_k_j_acc_valid) -> [rn_k_j_Acc_Valid]
  [Input_A_j_Read_Valid1] -> Input Memory Controller/6(Input_A_j_Read_Valid1)
  [Input_A_j_Read_Address1] -> Input Memory Controller/7(Input_A_j_Read_Address1)
  Mux Delay1/1 -> Memory Delay4/1
  Mux Delay2/1 -> Memory Delay3/1
  Mux Delay4/1 -> Memory Delay9/1
  Mux Delay5/1 -> Memory Delay10/1
  [A_k_Read_Valid1] -> A_k Memory Controller/4(A_k_Read_Valid1)
  [A_k_Read_Address1] -> A_k Memory Controller/5(A_k_Read_Address1)
  [Input_A_k_Read_Valid] -> Mem Address Select Delay6/1
  Mem Address Select Delay6/1 -> Memory Delay1/1
  Mem Address Select Delay7/1 -> Memory Delay7/1
  [Input_A_j_Read_Valid1] -> Mem Address Select Delay7/1
  Memory Delay1/1 -> Data Mux/3(r2_k_k_valid_in), Data_Mux_Valid_Or/1
  Memory Delay7/1 -> Data Mux/4(rn_k_j_valid_in), Data_Mux_Valid_Or/2
  Data_Mux_Valid_Or/1 -> Data Mux/1(Valid In)
  Const7/1 -> Data Mux/2(Channel In)
  [Input_Memory_Read_Data] -> Data Mux/7(Input_Memory_Read_Data)
  [A_k_Memory_Read_Data] -> Data Mux/8(A_k_Memory_Read_Data)
  Memory Delay9/1 -> Data Mux/11(Dot_Product_Acc_Init_In)
  Memory Delay10/1 -> Data Mux/12(r2_k_k_Acc_Valid_In)
  [rn_k_j_Acc_Valid] -> Mem Address Select Delay11/1
  Mem Address Select Delay11/1 -> Memory Delay11/1
  Memory Delay11/1 -> Data Mux/13(rn_k_j_Acc_Valid_In)
  Data Mux/2(Data Out 1) -> Dot Product/3(Data_In1)
  Data Mux/1(Valid Out) -> Dot Product/1(Valid_In)
  Data Mux/6(rn_k_j_Acc_Valid_Out) -> Dot Product/7(rn_k_j_valid_in)
  Const4/1 -> Inv SQRT/2(Channel In)
  Inv SQRT/2(inv_r_k_k) -> [inv_r_k_k]
  [inv_r2_k_k_valid_latch] -> Control Logic/5(inv_r2_k_k valid)
  Dot Product/4(rn_k_j_valid_out) -> rn_k_j SRlatch/1
  Const2/1 -> rn_k_j_over_r2_k_k/2(Channel In)
  Inv SQRT/4(inv_r2_k_k) -> rn_k_j_over_r2_k_k/4(inv_r2_k_k)
  rn_k_j_over_r2_k_k FIFO/1 -> [rn_k_j_over_r2_k_k_valid_latch]
  rn_k_j_over_r2_k_k FIFO/2 -> [rn_k_j_over_r2_k_k_data]
  A_j/2(A_j_Data_Out) -> [Aj_Feedback_Write_Data]
  rn_k_j_over_r2_k_k/1(Valid_out) -> rn_k_j_over_r2_k_k FIFO/1
  rn_k_j_over_r2_k_k/2(rn_k_j_over_r2_k_k) -> rn_k_j_over_r2_k_k FIFO/2
  [rn_k_j_over_r2_k_k_valid_latch] -> Control Logic/6(rn_k_j_over_r2_k_k valid)
  Control Logic/15(A_j_update_last_valid) -> [A_j_update_last_valid]
  Control Logic/14(A_k_Read_Address2) -> [A_k_Read_Address2]
  Control Logic/13(Input_A_j_Read_Address2) -> [Input_A_j_Read_Address2]
  Control Logic/12(Input_A_j_Read_Valid2) -> [A_k_Read_Valid2], [Input_A_j_Read_Valid2]
  [A_k_Read_Valid2] -> A_k Memory Controller/6(A_k_Read_Valid2)
  [A_k_Read_Address2] -> A_k Memory Controller/7(A_k_Read_Address2)
  [Input_A_j_Read_Valid2] -> Input Memory Controller/8(Input_A_j_Read_Valid2)
  [Input_A_j_Read_Address2] -> Input Memory Controller/9(Input_A_j_Read_Address2)
  Mem Address Select Delay8/1 -> Memory Delay8/1
  [Input_A_j_Read_Valid2] -> Mem Address Select Delay8/1
  Memory Delay8/1 -> Data Mux/5(A_j_update_valid_in), Data_Mux_Valid_Or/3
  [Input_A_j_Read_Address2] -> Mem Address Select Delay1/1
  Memory Delay2/1 -> Data Mux/14(A_j_Address_In)
  Mem Address Select Delay1/1 -> Memory Delay2/1
  [rn_k_j_over_r2_k_k_data] -> ExpandScalar/1
  ExpandScalar/1 -> Data Mux/9(rn_k_j_over_r2_k_k_fifo_Data)
  Data Mux/3(Data Out 2) -> Dot Product/4(Data_In2)
  Data Mux/5(r2_k_k_Acc_Valid_Out) -> Dot Product/6(r2_k_k_valid_in)
  Const13/1 -> A_j/2(Channel In)
  A_j/1(Valid_out) -> [Aj_Feedback_Write_Valid]
  A_j/3(Aj_Address_Out) -> [Aj_Feedback_Write_Address]
  Dot Product/6(Mult Data_out) -> A_j/3(Mult_Data_In), [Q_k_data]
  Data Mux/10(A_j_Address_Out) -> Dot Product/11(A_j_Address_In)
  Data Mux/9(Input_Memory_Read_Data_Out) -> Dot Product/10(A_j_Read_Data_In)
  Dot Product/10(A_j_Address_Out) -> A_j/5(Aj_Address_In)
  Dot Product/9(A_j_Read_Data_Out) -> A_j/4(A_j_Data_In)
  Data Mux/11(A_j_Update_last_Valid_Out) -> Dot Product/12(A_j_Update_last_Valid_In)
  Dot Product/11(A_j_Update_last_Valid_Out) -> A_j/6(A_j_Update_last_Valid_In)
  Memory Delay12/1 -> rn_k_j_over_r2_k_k FIFO/3
  [Aj_update_last_valid] -> Control Logic/7(Aj_update_last_valid)
  Data Mux/7(A_j_update_valid_Out) -> Dot Product/8(A_j_update_valid_in)
  Dot Product/2(Dot Product Data_Out) -> rk/3(rn_k_j), rn_k_j_over_r2_k_k/3(rn_k_j), Inv SQRT/3(r2_k_k)
  A_j/4(A_j_Update_last_Valid_Out) -> [Aj_update_last_valid]
  [Aj_Feedback_Write_Valid] -> Feedback delay/1
  [Aj_Feedback_Write_Data] -> Feedback delay2/1
  [Aj_Feedback_Write_Address] -> Feedback delay1/1
  Feedback delay/1 -> Input Memory Controller/10(Feedback Write)
  Feedback delay1/1 -> Input Memory Controller/11(Feedback Address)
  Feedback delay2/1 -> Input Memory Controller/12(Feedback Data)
  Const5/1 -> rk/2(Channel In)
  rk/1(Valid_out) -> [r_k_j_valid]
  rk/2(r_k_j) -> [r_k_j_data]
  [inv_r_k_k] -> rk/4(inv_r_k_k)
  Control Logic/17(A_k_Read_Valid3) -> [A_k_Read_Valid3]
  Control Logic/18(A_k_Read_Address3) -> [A_k_Read_Address3]
  [A_k_Read_Valid3] -> A_k Memory Controller/8(A_k_Read_Valid3)
  [A_k_Read_Address3] -> A_k Memory Controller/9(A_k_Read_Address3)
  Mem Address Select Delay3/1 -> Memory Delay6/1
  [A_k_Read_Valid3] -> Mem Address Select Delay3/1
  Memory Delay6/1 -> Data Mux/6(Q_k_valid_in), Data_Mux_Valid_Or/4
  Const11/1 -> Real-Imag to Complex/2
  ExpandScalar1/1 -> Data Mux/10(inv_r_k_k_Data)
  Real-Imag to Complex/1 -> ExpandScalar1/1
  Data Mux/8(Q_k_valid_Out) -> Dot Product/9(Q_k_valid_in)
  Dot Product/7(A_j_update_valid_Out) -> A_j/1(Valid In)
  Dot Product/8(Q_k_valid_Out) -> [Q_k_valid]
  [inv_r_k_k] -> Mux Delay3/1
  Mux Delay3/1 -> Real-Imag to Complex/1
  [A_j_update_last_valid] -> Mem Address Select Delay12/1
  Mem Address Select Delay12/1 -> Memory Delay12/1
  Memory Delay5/1 -> Data Mux/15(A_j_Update_last_Valid_In)
  Mem Address Select Delay2/1 -> Memory Delay5/1
  [A_j_update_last_col_valid] -> Mem Address Select Delay2/1
  Control Logic/16(A_j_update_last_col_valid) -> [A_j_update_last_col_valid]
  Control Logic/20(Done) -> [Control_Done]
  Memory Delay13/1 -> Data Mux/16(Done_In)
  Mem Address Select Delay4/1 -> Memory Delay13/1
  [Control_Done] -> Mem Address Select Delay4/1
  Data Mux/12(Done_Out) -> Dot Product/13(Done_In)
  Dot Product/12(Done_Out) -> A_j/7(Done_In)
  A_j/5(Done_Out) -> [QRD_Done]
  [Q_k_data] -> Q Output Memory Controller/2(Write Data)
  [Q_k_valid] -> Q Output Memory Controller/1(Write Enable)
  [Control_Start] -> Q Output Memory Controller/3(Wr_Addr_Clr)
  [inv_r_k_k] -> Inv_Rk Output Memory Controller/2(Write Data)
  [inv_r_k_k_valid] -> Inv_Rk Output Memory Controller/1(Write Enable)
  [Control_Start] -> Inv_Rk Output Memory Controller/3(Wr_Addr_Clr)
  Inv SQRT/1(inv_r_k_k_valid_out) -> [inv_r_k_k_valid]
  [r_k_j_data] -> Rn Output Memory Controller/2(Write Data)
  [r_k_j_valid] -> Rn Output Memory Controller/1(Write Enable)
  [Control_Start] -> Rn Output Memory Controller/3(Wr_Addr_Clr)
  [QRD_Done] -> Q Output Memory Controller/4(Done)
  [size] -> Q Output Memory Controller/6(Size)
  [size] -> Inv_Rk Output Memory Controller/6(Size)
  [QRD_Done] -> Inv_Rk Output Memory Controller/4(Done)
  [QRD_Done] -> Rn Output Memory Controller/4(Done)
  [size] -> Rn Output Memory Controller/6(Size)
  Q Source Ready/1 -> Q Output Memory Controller/5(Source Ready)
  Latch/3 -> [Channel_Out]
  [Channel_Out] -> Channel Latch/3
  Const8/1 -> Channel Latch/2
  [QRD_Done] -> Channel Latch/1
  Channel Latch/3 -> Q Source Channel/1, Inv Rk Source Channel/1, Rn Source Channel/1
  Q Output Memory Controller/1(Source Valid) -> Q Source Valid/1
  Q Output Memory Controller/2(Source Data) -> Q Source Data/1
  Q Output Memory Controller/3(Source SOP) -> Q Source SOP/1
  Q Output Memory Controller/4(Source EOP) -> Q Source EOP/1
  Q Output Memory Controller/5(Output_Busy) -> [Q_Output_Busy]
  Inv_Rk Output Memory Controller/1(Source Valid) -> Inv Rk Source Valid/1
  Inv_Rk Output Memory Controller/2(Source Data) -> Inv Rk Source Data/1
  Inv_Rk Output Memory Controller/3(Source SOP) -> Inv Rk Source SOP/1
  Inv_Rk Output Memory Controller/4(Source EOP) -> Inv Rk Source EOP/1
  Inv_Rk Output Memory Controller/5(Output_Busy) -> [Inv_Rk_Output_Busy]
  Inv Rk Source Ready/1 -> Inv_Rk Output Memory Controller/5(Source Ready)
  Rn Source Ready/1 -> Rn Output Memory Controller/5(Source Ready)
  Rn Output Memory Controller/1(Source Valid) -> Rn Source Valid/1
  Rn Output Memory Controller/2(Source Data) -> Rn Source Data/1
  Rn Output Memory Controller/3(Source SOP) -> Rn Source SOP/1
  Rn Output Memory Controller/4(Source EOP) -> Rn Source EOP/1
  Rn Output Memory Controller/5(Output_Busy) -> [Rn_Output_Busy]
  [Q_Output_Busy] -> Or/1
  [Inv_Rk_Output_Busy] -> Or/2
  [Rn_Output_Busy] -> Or/3
  Inv SQRT/3(inv_r2_k_k_valid_out) -> inv_r2_k_k SRlatch/1
  [Column_Done] -> inv_r2_k_k SRlatch/2
  Control Logic/19(Column_Done) -> [Column_Done]
  inv_r2_k_k SRlatch/1 -> [inv_r2_k_k_valid_latch]
  And4/1 -> Rising Edge Detect3/1
  rn_k_j SRlatch/1 -> And4/1, And/1
  [inv_r2_k_k_valid_latch] -> Not2/1, And4/2
  Rising Edge Detect3/1 -> rn_k_j SRlatch/2, rk/1(Valid In), rn_k_j_over_r2_k_k/1(Valid In)
  Not2/1 -> And/2
  And/1 -> [rn_k_j_backpressure]
  Not3/1 -> Control Logic/8(rn_k_j_loop_enable)
  [rn_k_j_backpressure] -> Not3/1
